simulink model "q2_e"  (R2016a)
settings: Solver=VariableStepAuto  StartTime=0.0  StopTime=10.0  RelTol=1e-3
settings Model: Creator=Huang Shemin  LastModifiedBy=Huang Shemin

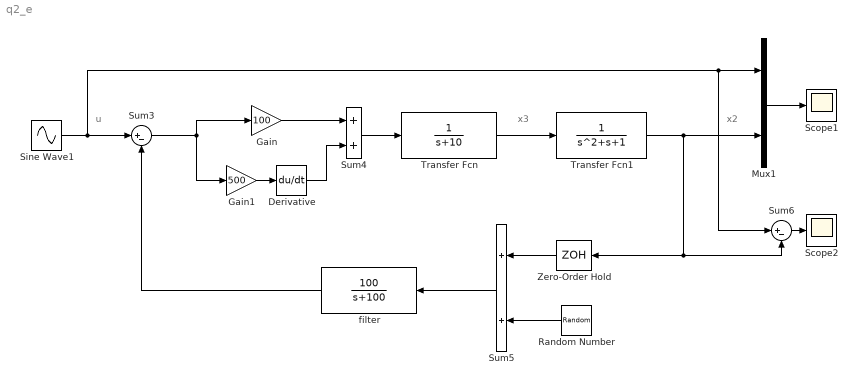
== system q2_e ==
  note: x2
  note: x3
  note: u
  Derivative : Derivative
  Gain : Gain  Gain=100
  Gain1 : Gain  Gain=500
  Mux1 : Mux  Inputs=2
  Random Number : RandomNumber  Variance=0.01  SampleTime=0.005
  Scope1 : Scope
  Scope2 : Scope
  Sine Wave1 : Sin  Frequency=2*pi  SampleTime=0
  Sum3 : Sum  Inputs=|+-
  Sum4 : Sum
  Sum5 : Sum
  Sum6 : Sum  Inputs=|+-
  Transfer Fcn : TransferFcn  Denominator=[1 10]
  Transfer Fcn1 : TransferFcn  Denominator=[1 1 1]
  Zero-Order Hold : ZeroOrderHold  SampleTime=0.005
  filter : TransferFcn  Numerator=[100]  Denominator=[1 100]
  wires:
  Transfer Fcn/1 -> Transfer Fcn1/1
  Sine Wave1/1 -> Sum6/1, Mux1/1, Sum3/1
  Mux1/1 -> Scope1/1
  Transfer Fcn1/1 -> Mux1/2, Sum6/2, Zero-Order Hold/1
  Zero-Order Hold/1 -> Sum5/1
  Sum4/1 -> Transfer Fcn/1
  Sum3/1 -> Gain/1, Gain1/1
  Random Number/1 -> Sum5/2
  Sum5/1 -> filter/1
  filter/1 -> Sum3/2
  Gain1/1 -> Derivative/1
  Derivative/1 -> Sum4/2
  Gain/1 -> Sum4/1
  Sum6/1 -> Scope2/1
